simulink subsystem "subsystem_desiredMotorTrajectory"  (R2022a)
settings: Solver=VariableStepAuto  StartTime=0.0  StopTime=10.0  RelTol=1e-3
settings Model: Creator=ge75qet  LastModifiedBy=Philipp

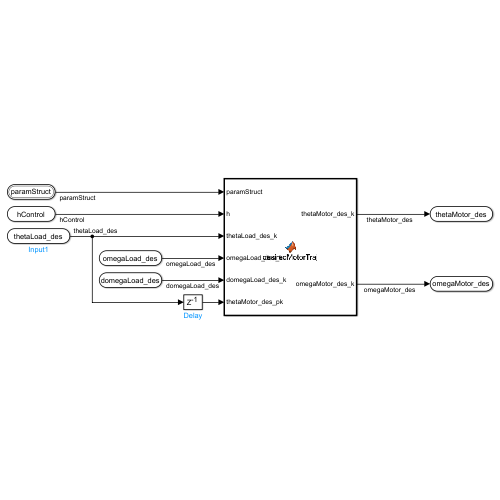
[thumbnail: Simulink's stored preview of the top-level diagram]
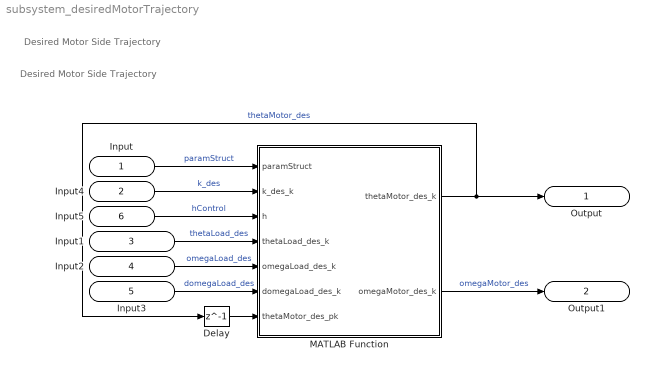
== system subsystem_desiredMotorTrajectory ==
  note: Desired Motor Side Trajectory
  note: Desired Motor Side Trajectory
  Input : Inport  OutDataTypeStr=Bus: main_bus
  Input4 : Inport  Port=2
  Input1 : Inport  Port=3
  Input2 : Inport  Port=4
  Input3 : Inport  Port=5
  Input5 : Inport  Port=6
  Delay : Delay  DelayLength=1
  MATLAB Function : MATLAB Function  TreatAsAtomicUnit=on
  Output : Outport
  Output1 : Outport  Port=2
  wires:
  Input4/1 -> MATLAB Function/2(k_des_k)  "k_des"
  Delay/1 -> MATLAB Function/7(thetaMotor_des_pk)
  MATLAB Function/2(omegaMotor_des_k) -> Output1/1  "omegaMotor_des"
  Input3/1 -> MATLAB Function/6(domegaLoad_des_k)  "domegaLoad_des"
  MATLAB Function/1(thetaMotor_des_k) -> Delay/1, Output/1  "thetaMotor_des"
  Input1/1 -> MATLAB Function/4(thetaLoad_des_k)  "thetaLoad_des"
  Input2/1 -> MATLAB Function/5(omegaLoad_des_k)  "omegaLoad_des"
  Input/1 -> MATLAB Function/1(paramStruct)  "paramStruct"
  Input5/1 -> MATLAB Function/3(h)  "hControl"

== matlab function subsystem_desiredMotorTrajectory/MATLAB Function ==
  data: paramStruct input; k_des_k input; thetaMotor_des_k output; h input; thetaLoad_des_k input; omegaLoad_des_k input; domegaLoad_des_k input; thetaMotor_des_pk input; omegaMotor_des_k output
function [thetaMotor_des_k, omegaMotor_des_k] = desiredMotorTraj(paramStruct, k_des_k, h, thetaLoad_des_k, omegaLoad_des_k, domegaLoad_des_k, thetaMotor_des_pk)

[thetaMotor_des_k, omegaMotor_des_k] = ...
    desiredMotorTraj_fun(paramStruct, k_des_k, h, thetaLoad_des_k, omegaLoad_des_k, domegaLoad_des_k, thetaMotor_des_pk);
